simulink model "sampleModel1974"  (R2023a)
settings: Solver=VariableStepAuto  StartTime=0.0  StopTime=10.0  RelTol=1e-3
libraries: simulink x3, hdlsllib x3
settings Model: Creator=user1  LastModifiedBy=user1

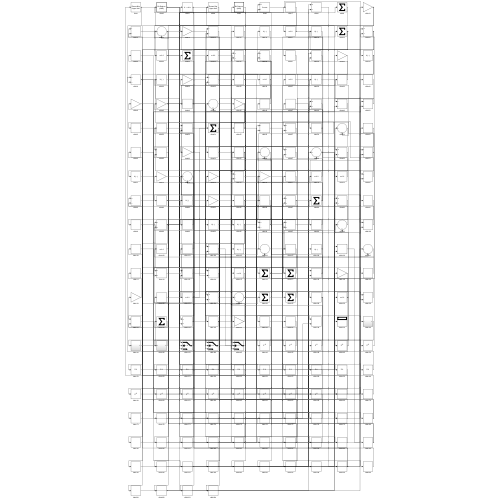
[thumbnail: Simulink's stored preview of the top-level diagram]
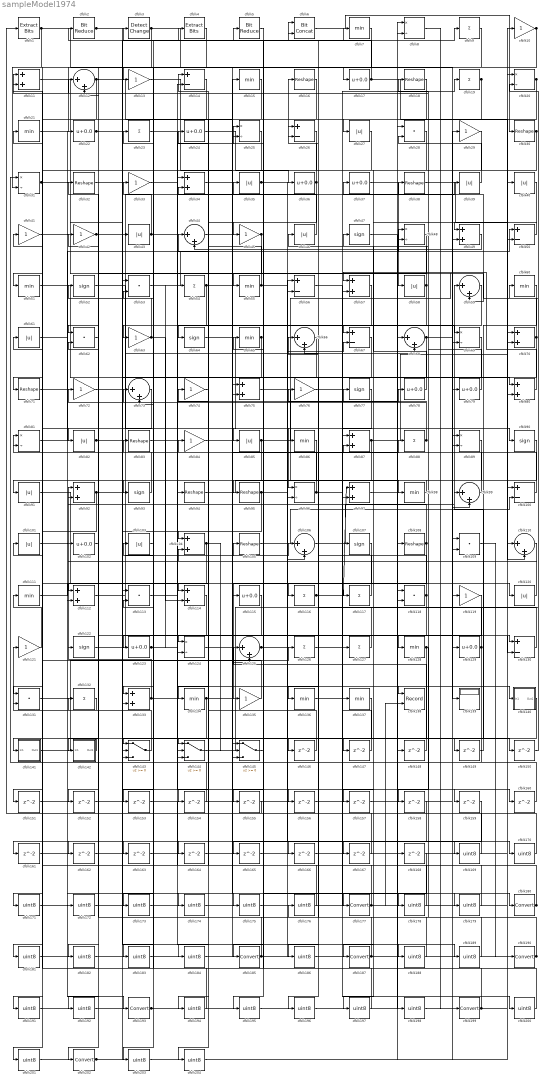
== system sampleModel1974 ==
  cfblk1 : simulink/Logic and Bit Operations/Extract Bits  bitsToExtract=Upper half  numBits=8  bitIdxRange=[0 7]  outScalingMode=Preserve fixed-point scaling
      settings: LibrarySourceBlock=|
      | hdlsllib/Logic and Bit
      | Operations/Extract Bits
  cfblk{10,13,29,33,41..42,45,63,72,74,76,84,119,121,135} (15 alike) : Gain
  cfblk{14,26,50,56,67,100,130} (7 alike) : Sum  Inputs=+-
  cfblk{27,35,39..40,43,46,58,61,82,85,91,101,103,120} (14 alike) : Abs  SaturateOnIntegerOverflow=off
  cfblk{17,22,24,36..37,78..79,102,115,123,129} (11 alike) : Bias  Bias=0.0  SaturateOnIntegerOverflow=off
  cfblk{11,34,49,57,70,75,80,87,92,97,104,112,114,133} (14 alike) : Sum
  cfblk{16,18,30,32,38,71,83,94..95,105,108} (11 alike) : Reshape
  cfblk{12,44,59,66,68,73,99,106,110,125} (10 alike) : Sum  Inputs=|++
  cfblk{47,52,64,77,90,93,107,122} (8 alike) : Signum
  cfblk{28,53,62,109,113,118,131} (7 alike) : DotProduct  OutDataTypeStr=Inherit: Inherit via internal rule
  cfblk{7,15,21,51,55,60,65,86,98,111,128,134,136..137} (14 alike) : MinMax
  cfblk{9,19,23,54,88,116..117,126..127,132} (10 alike) : Sum  Inputs=+
  cfblk{8,20,25,31,48,69,81,89,96,124} (10 alike) : Product  Inputs=*/  RndMeth=Zero  SaturateOnIntegerOverflow=on
  cfblk138 : Record  FileSettingsInternal="{\"entries\":[{\"content\":{\"excelSettings\":{\"content\":{},\"type\":\"Streamout.ExcelSettings\"}},\"type\":\"Streamout.FileSettingStorage\",\"uuid\":\"\"}],\"packageUris\":[\"http:\\/\\/schema.mathworks.com\\/mf0\\/streamout_blocks\\/R2020a\"],\"version\":\"1.0\"}"  Layout=[1 1]  SignalsInternal="{\"entries\":[{\"content\":{\"signals\":[{\"content\":{\"blockPath\":[],\"dimensions\":[1],\"domain\":\"\",\"lineColor\":\"#a2142f\",\"plots\":[1],\"port\":1,\"signalID\":5620,\"signalName\":\"XY Graph:1\"},\"type\":\"RecordBlkView.Signal\",\"uuid\":\"\"},{\"content\":{\"blockPath\":[],\"dimensions\":[1],\"domain\":\"\",\"lineColor\":\"#139fff\",\"plots\":[1],\"port\":2,\"signalID\":5623,\"signalName\":\"XY Graph:2\"},\"type\":\"RecordBlkView.Signal\",\"uuid\":\"\"}]},\"type\":\"RecordBlkView.InputSignals\",\"uuid\":\"\"}],\"packageUris\":[\"http:\\/\\/schema.mathworks.com\\/mf0\\/streamout_blocks\\/R2020a\"],\"version\":\"1.0\"}"  VisualizationBindings="{\"xyplotplugin\":{\"info\":[{\"series\":[{\"bindingParametersList\":[{\"parameter\":\"X-Axis\",\"signalID\":5620,\"signalName\":\"XY Graph:1\"},{\"parameter\":\"Y-Axis\",\"signalID\":5623,\"signalName\":\"XY Graph:2\"}],\"seriesID\":47147}],\"subplotID\":1}]}}"  CompatibilityTag=XY  st=-1
  cfblk139 : Display
  cfblk140 : Subsystem
      settings: LibrarySourceBlock=|
      | hdlsllib/Ports &
      | Subsystems/Subsystem
  cfblk141 : Subsystem
      settings: LibrarySourceBlock=|
      | hdlsllib/Ports &
      | Subsystems/Subsystem
  cfblk142 : Subsystem
      settings: LibrarySourceBlock=|
      | hdlsllib/Ports &
      | Subsystems/Subsystem
  cfblk143 : Switch  SaturateOnIntegerOverflow=off  InputSameDT=off
  cfblk144 : Switch  SaturateOnIntegerOverflow=off  InputSameDT=off
  cfblk145 : Switch  SaturateOnIntegerOverflow=off  InputSameDT=off
  cfblk{146..168} (23 alike) : Delay  SampleTime=1
  cfblk{169..176,178..179,181..184,186,188..189,191..192,194..198,200..201,203..204} (28 alike) : DataTypeConversion  OutDataTypeStr=uint8  SaturateOnIntegerOverflow=off  RndMeth=Floor
  cfblk{177,180,185,187,190,193,199,202} (8 alike) : DataTypeConversion  SaturateOnIntegerOverflow=off  RndMeth=Floor
  cfblk2 : hdlsllib/Logic and Bit Operations/Bit Reduce  mode=AND
  cfblk3 : simulink/Logic and Bit Operations/Detect Change  vinit=0  OutDataTypeStr=boolean
      settings: LibrarySourceBlock=|
      | hdlsllib/Logic and Bit
      | Operations/Detect
      | Change
  cfblk4 : simulink/Logic and Bit Operations/Extract Bits  bitsToExtract=Upper half  numBits=8  bitIdxRange=[0 7]  outScalingMode=Preserve fixed-point scaling
      settings: LibrarySourceBlock=|
      | hdlsllib/Logic and Bit
      | Operations/Extract Bits
  cfblk5 : hdlsllib/Logic and Bit Operations/Bit Reduce  mode=AND
  cfblk6 : hdlsllib/Logic and Bit Operations/Bit Concat  numInputs=2
  wires:
  cfblk94/1 -> cfblk98/1
  cfblk122/1 -> cfblk35/1
  cfblk106/1 -> cfblk59/1
  cfblk52/1 -> cfblk85/1
  cfblk56/1 -> cfblk180/1
  cfblk85/1 -> cfblk59/2, cfblk123/1
  cfblk80/1 -> cfblk57/1
  cfblk133/1 -> cfblk92/1, cfblk78/1
  cfblk65/1 -> cfblk143/3, cfblk203/1
  cfblk43/1 -> cfblk33/1, cfblk80/1, cfblk140/1(In1)
  cfblk99/1 -> cfblk81/1
  cfblk78/1 -> cfblk47/1
  cfblk58/1 -> cfblk6/2, cfblk184/1
  cfblk116/1 -> cfblk97/1, cfblk39/1
  cfblk62/1 -> cfblk112/1
  cfblk144/1 -> cfblk60/1
  cfblk134/1 -> cfblk143/1, cfblk88/1
  cfblk50/1 -> cfblk49/1
  cfblk36/1 -> cfblk16/1, cfblk164/1, cfblk165/1
  cfblk91/1 -> cfblk117/1
  cfblk73/1 -> cfblk91/1
  cfblk34/1 -> cfblk177/1
  cfblk82/1 -> cfblk68/2, cfblk145/3
  cfblk42/1 -> cfblk38/1, cfblk174/1
  cfblk9/1 -> cfblk17/1
  cfblk129/1 -> cfblk31/1, cfblk48/2
  cfblk64/1 -> cfblk96/1
  cfblk46/1 -> cfblk14/1
  cfblk145/1 -> cfblk65/1
  cfblk29/1 -> cfblk95/1
  cfblk14/1 -> cfblk71/1
  cfblk49/1 -> cfblk44/2
  cfblk7/1 -> cfblk51/1
  cfblk75/1 -> cfblk127/1
  cfblk6/1 -> cfblk30/1
  cfblk28/1 -> cfblk187/1
  cfblk8/1 -> cfblk199/1
  cfblk24/1 -> cfblk36/1
  cfblk100/1 -> cfblk23/1
  cfblk27/1 -> cfblk45/1
  cfblk12/1 -> cfblk75/1, cfblk191/1, cfblk192/1
  cfblk126/1 -> cfblk107/1
  cfblk119/1 -> cfblk185/1
  cfblk89/1 -> cfblk202/1
  cfblk98/1 -> cfblk93/1
  cfblk96/1 -> cfblk19/1, cfblk73/1
  cfblk132/1 -> cfblk121/1
  cfblk17/1 -> cfblk100/1, cfblk2/1
  cfblk54/1 -> cfblk63/1, cfblk138/1
  cfblk88/1 -> cfblk72/1, cfblk26/2
  cfblk44/1 -> cfblk69/1
  cfblk103/1 -> cfblk83/1
  cfblk5/1 -> cfblk55/1
  cfblk121/1 -> cfblk111/1
  cfblk51/1 -> cfblk94/1
  cfblk3/1 -> cfblk99/2, cfblk12/2
  cfblk107/1 -> cfblk135/1
  cfblk77/1 -> cfblk97/2
  cfblk141/1(Out1) -> cfblk126/1
  cfblk20/1 -> cfblk82/1, cfblk27/1
  cfblk135/1 -> cfblk101/1
  cfblk102/1 -> cfblk52/1
  cfblk130/1 -> cfblk26/1
  cfblk109/1 -> cfblk190/1
  cfblk105/1 -> cfblk100/2
  cfblk128/1 -> cfblk157/1, cfblk158/1
  cfblk117/1 -> cfblk46/1
  cfblk2/1 -> cfblk128/1, cfblk159/1, cfblk160/1
  cfblk92/1 -> cfblk4/1, cfblk116/1, cfblk9/1, cfblk161/1
  cfblk68/1 -> cfblk136/1, cfblk130/2, cfblk90/1
  cfblk45/1 -> cfblk62/1, cfblk64/1
  cfblk41/1 -> cfblk112/2
  cfblk72/1 -> cfblk139/1
  cfblk87/1 -> cfblk20/1, cfblk143/2
  cfblk32/1 -> cfblk7/1
  cfblk97/1 -> cfblk130/1
  cfblk11/1 -> cfblk79/1
  cfblk142/1(Out1) -> cfblk141/1(In1)
  cfblk10/1 -> cfblk22/1, cfblk13/1
  cfblk66/1 -> cfblk104/1
  cfblk81/1 -> cfblk50/1
  cfblk30/1 -> cfblk151/1, cfblk152/1
  cfblk143/1 -> cfblk132/1
  cfblk112/1 -> cfblk106/1
  cfblk39/1 -> cfblk18/1
  cfblk93/1 -> cfblk42/1
  cfblk61/1 -> cfblk193/1
  cfblk67/1 -> cfblk124/1
  cfblk55/1 -> cfblk11/1, cfblk147/1
  cfblk108/1 -> cfblk73/2, cfblk166/1
  cfblk13/1 -> cfblk145/1
  cfblk19/1 -> cfblk114/1, cfblk182/1
  cfblk31/1 -> cfblk113/1, cfblk150/1
  cfblk69/1 -> cfblk96/2
  cfblk48/1 -> cfblk144/1
  cfblk79/1 -> cfblk12/1
  cfblk83/1 -> cfblk25/1
  cfblk33/1 -> cfblk67/1
  cfblk35/1 -> cfblk115/1, cfblk167/1
  cfblk111/1 -> cfblk120/1
  cfblk57/1 -> cfblk133/1
  cfblk123/1 -> cfblk105/1, cfblk54/1
  cfblk104/1 -> cfblk131/1, cfblk145/2
  cfblk63/1 -> cfblk32/1, cfblk114/2
  cfblk113/1 -> cfblk14/2
  cfblk114/1 -> cfblk124/2
  cfblk127/1 -> cfblk76/1
  cfblk1/1 -> cfblk125/2, cfblk31/2
  cfblk118/1 -> cfblk92/2, cfblk144/3, cfblk102/1
  cfblk95/1 -> cfblk77/1, cfblk133/2, cfblk204/1
  cfblk38/1 -> cfblk110/2
  cfblk74/1 -> cfblk134/1
  cfblk37/1 -> cfblk58/1
  cfblk115/1 -> cfblk142/1(In1)
  cfblk71/1 -> cfblk48/1
  cfblk22/1 -> cfblk6/1, cfblk189/1
  cfblk110/1 -> cfblk104/2
  cfblk53/1 -> cfblk29/1
  cfblk125/1 -> cfblk87/2, cfblk67/2
  cfblk120/1 -> cfblk24/1
  cfblk70/1 -> cfblk144/2, cfblk37/1
  cfblk124/1 -> cfblk146/1
  cfblk146/1 -> cfblk44/1
  cfblk147/1 -> cfblk87/1
  cfblk148/1 -> cfblk125/1
  cfblk60/1 -> cfblk149/1
  cfblk149/1 -> cfblk99/1
  cfblk150/1 -> cfblk20/2
  cfblk151/1 -> cfblk49/2
  cfblk152/1 -> cfblk75/2
  cfblk4/1 -> cfblk153/1
  cfblk26/1 -> cfblk154/1
  cfblk154/1 -> cfblk81/2
  cfblk18/1 -> cfblk155/1
  cfblk155/1 -> cfblk1/1
  cfblk23/1 -> cfblk156/1
  cfblk156/1 -> cfblk57/2
  cfblk157/1 -> cfblk69/2
  cfblk160/1 -> cfblk66/2
  cfblk161/1 -> cfblk80/2
  cfblk25/1 -> cfblk162/1
  cfblk162/1 -> cfblk53/1
  cfblk16/1 -> cfblk163/1
  cfblk164/1 -> cfblk50/2
  cfblk165/1 -> cfblk106/2
  cfblk166/1 -> cfblk118/2
  cfblk167/1 -> cfblk11/2
  cfblk84/1 -> cfblk169/1
  cfblk169/1 -> cfblk41/1
  cfblk76/1 -> cfblk170/1
  cfblk170/1 -> cfblk84/1
  cfblk86/1 -> cfblk171/1
  cfblk171/1 -> cfblk118/1
  cfblk101/1 -> cfblk172/1
  cfblk172/1 -> cfblk86/1
  cfblk137/1 -> cfblk173/1
  cfblk173/1 -> cfblk108/1
  cfblk174/1 -> cfblk137/1
  cfblk21/1 -> cfblk175/1
  cfblk175/1 -> cfblk110/1
  cfblk176/1 -> cfblk21/1
  cfblk177/1 -> cfblk74/1, cfblk138/2, cfblk53/2
  cfblk131/1 -> cfblk178/1
  cfblk178/1 -> cfblk34/1
  cfblk153/1 -> cfblk179/1
  cfblk179/1 -> cfblk34/2
  cfblk180/1 -> cfblk131/2, cfblk5/1
  cfblk158/1 -> cfblk181/1
  cfblk181/1 -> cfblk56/1
  cfblk182/1 -> cfblk56/2
  cfblk15/1 -> cfblk183/1
  cfblk183/1 -> cfblk129/1
  cfblk184/1 -> cfblk15/1
  cfblk185/1 -> cfblk113/2, cfblk70/1
  cfblk140/1(Out1) -> cfblk186/1
  cfblk186/1 -> cfblk119/1
  cfblk187/1 -> cfblk176/1, cfblk66/1
  cfblk163/1 -> cfblk188/1
  cfblk188/1 -> cfblk28/1
  cfblk189/1 -> cfblk28/2
  cfblk190/1 -> cfblk62/2, cfblk122/1
  cfblk191/1 -> cfblk109/1
  cfblk192/1 -> cfblk109/2
  cfblk193/1 -> cfblk148/1, cfblk10/1
  cfblk59/1 -> cfblk194/1
  cfblk194/1 -> cfblk61/1
  cfblk168/1 -> cfblk195/1
  cfblk195/1 -> cfblk68/1
  cfblk90/1 -> cfblk196/1
  cfblk196/1 -> cfblk168/1
  cfblk40/1 -> cfblk197/1
  cfblk197/1 -> cfblk103/1
  cfblk47/1 -> cfblk198/1
  cfblk198/1 -> cfblk40/1
  cfblk199/1 -> cfblk25/2, cfblk3/1
  cfblk136/1 -> cfblk200/1
  cfblk200/1 -> cfblk8/1
  cfblk159/1 -> cfblk201/1
  cfblk201/1 -> cfblk8/2
  cfblk202/1 -> cfblk43/1, cfblk70/2
  cfblk203/1 -> cfblk89/1
  cfblk204/1 -> cfblk89/2

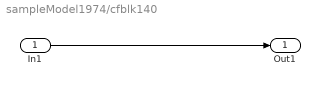
== system sampleModel1974/cfblk140 ==
  In1 : Inport
  Out1 : Outport
  wires:
  In1/1 -> Out1/1

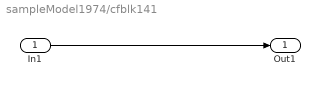
== system sampleModel1974/cfblk141 ==
  In1 : Inport
  Out1 : Outport
  wires:
  In1/1 -> Out1/1

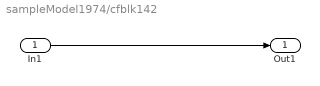
== system sampleModel1974/cfblk142 ==
  In1 : Inport
  Out1 : Outport
  wires:
  In1/1 -> Out1/1
